simulink library "halin"  (R2021b)
settings: Solver=VariableStepAuto  StartTime=0.0  StopTime=10.0  RelTol=1e-3
undefined symbols (not defined in the file): KHAL_CAN1ABM1E2E_flg, KHAL_CAN1EPB1E2E_flg, KHAL_CAN1EPS1E2E_flg, KHAL_CAN1ESC1E2E_flg, KHAL_CAN1ESC5E2E_flg, KHAL_CAN3BMS1E2E_flg, KHAL_CAN3BMS6E2E_flg, KHAL_CAN3CCU1E2E_flg, KHAL_CAN3CCU2E2E_flg, KHAL_CAN3MCUNF1E2E_flg, KHAL_CAN3MCUNR1E2E_flg, KHAL_CAN3Shifter1E2E_flg, KHAL_CAN3Shifter2E2E_flg, KHAL_CAN6FCM2E2E_flg, KHAL_CAN6FCM4E2E_flg, TRUE
libraries: simulink x645, FVT_lib x207, hcu_lib x59
(part 1 of 23)
settings Model: Creator=13168  LastModifiedBy=FVT23033
settings SolverCC: AlgebraicLoopSolver=TrustRegion
settings DataIOCC: SaveFormat=Array  SignalLoggingSaveFormat=ModelDataLogs  ReturnWorkspaceOutputs=off
settings OptimizationCC: BlockReduction=off  BooleanDataType=off
settings DebuggingCC: SaveWithParameterizedLinksMsg=none  UnderspecifiedInitializationDetection=Classic  MergeDetectMultiDrivingBlocksExec=none  SignalResolutionControl=TryResolveAllWithWarning  SFMachineParentedDataDiag=warning
settings HardwareCC: TargetUnknown=on
settings ModelReferenceCC: PropagateSignalLabelsOutOfModel=off
settings ConfigComp: CovMetricSettings=dw  CovSaveCumulativeToWorkspaceVar=on  CovSaveSingleToWorkspaceVar=on

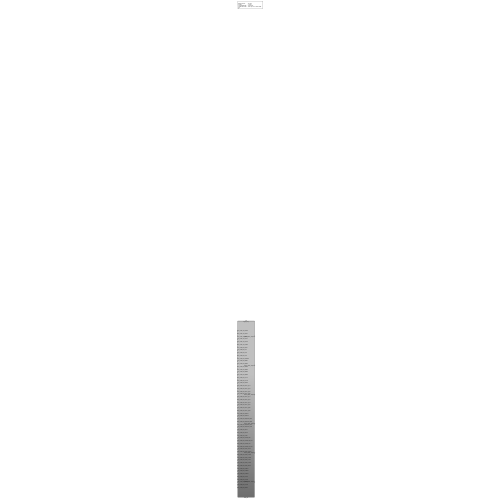
[thumbnail: Simulink's stored preview of the top-level diagram]
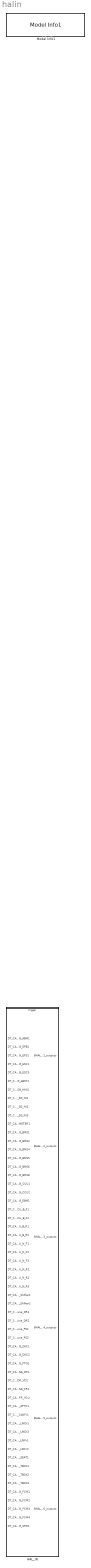
== system halin ==
  HAL_IN : Subsystem
      settings: RTWSystemCode=Nonreusable function  RTWFcnNameOpts=Use subsystem name  RTWFileNameOpts=Use subsystem name
  Model Info1 : hcu_lib/Model Info1  BlockCM=None  Frame=on  DisplayStringWithTags=|  HorizontalTextAlignment=Left  LeftAlignmentValue=0.02  SourceBlockDiagram=hcu_lib  TagMaxNumber=20
      | Model Version        : %<ModelVersion>
      | Creator                   : %<Creator>
      | Last Modified By    : %<LastModifiedBy>
      | Modification date    : %<LastModificationDate>
      settings: SourceProductName=HCU Relative Block Library

== system halin/HAL_IN ==
  DT_CAN1_SG_ABM1 : Inport
  DT_CAN1_SG_EPB1 : Inport  Port=2
  DT_CAN1_SG_EPS1 : Inport  Port=3
  DT_CAN1_SG_ESC1 : Inport  Port=4
  DT_CAN1_SG_ESC5 : Inport  Port=5
  DT_CAN1_SG_eBST1 : Inport  Port=6
  DT_CAN2_SG_HMI1 : Inport  Port=7
  DT_CAN2_SG_IVI1 : Inport  Port=8
  DT_CAN2_SG_IVI2 : Inport  Port=9
  DT_CAN2_SG_IVI3 : Inport  Port=10
  DT_CAN2_SG_METER1 : Inport  Port=11
  DT_CAN3_SG_BMS1 : Inport  Port=12
  DT_CAN3_SG_BMS3 : Inport  Port=13
  DT_CAN3_SG_BMS4 : Inport  Port=14
  DT_CAN3_SG_BMS5 : Inport  Port=15
  DT_CAN3_SG_BMS6 : Inport  Port=16
  DT_CAN3_SG_BMS8 : Inport  Port=17
  DT_CAN3_SG_CCU1 : Inport  Port=18
  DT_CAN3_SG_CCU2 : Inport  Port=19
  DT_CAN3_SG_EBM1 : Inport  Port=20
  DT_CAN3_SG_MCU_B_F1 : Inport  Port=21
  DT_CAN3_SG_MCU_B_F2 : Inport  Port=22
  DT_CAN3_SG_MCU_B_R1 : Inport  Port=23
  DT_CAN3_SG_MCU_B_R2 : Inport  Port=24
  DT_CAN3_SG_MCU_N_F1 : Inport  Port=25
  DT_CAN3_SG_MCU_N_F2 : Inport  Port=26
  DT_CAN3_SG_MCU_N_F3 : Inport  Port=27
  DT_CAN3_SG_MCU_N_R1 : Inport  Port=28
  DT_CAN3_SG_MCU_N_R2 : Inport  Port=29
  DT_CAN3_SG_MCU_N_R3 : Inport  Port=30
  DT_CAN3_SG_Shifter1 : Inport  Port=31
  DT_CAN3_SG_Shifter2 : Inport  Port=32
  DT_CAN4_SG_BodyZone_DR1 : Inport  Port=33
  DT_CAN4_SG_BodyZone_DR2 : Inport  Port=34
  DT_CAN4_SG_BodyZone_PS1 : Inport  Port=35
  DT_CAN4_SG_BodyZone_PS2 : Inport  Port=36
  DT_CAN4_SG_DKC1 : Inport  Port=37
  DT_CAN4_SG_DKC2 : Inport  Port=38
  DT_CAN4_SG_PTG1 : Inport  Port=39
  DT_CAN4_SG_ZONE_DR1 : Inport  Port=40
  DT_CAN4_SG_ZONE_DR_VCU : Inport  Port=41
  DT_CAN4_SG_ZONE_FR1 : Inport  Port=42
  DT_CAN4_SG_ZONE_FR_VCU : Inport  Port=43
  DT_CAN4_SG_zGW_APTC1 : Inport  Port=44
  DT_CAN4_SG_zGW_CANFr1 : Inport  Port=45
  DT_CAN4_SG_zGW_LINDr1 : Inport  Port=46
  DT_CAN4_SG_zGW_LINDr2 : Inport  Port=47
  DT_CAN4_SG_zGW_LINFr1 : Inport  Port=48
  DT_CAN4_SG_zGW_LINFr2 : Inport  Port=49
  DT_CAN4_SG_zGW_SEAT1 : Inport  Port=50
  DT_CAN5_SG_TBOX1 : Inport  Port=51
  DT_CAN5_SG_TBOX2 : Inport  Port=52
  DT_CAN5_SG_TBOX3 : Inport  Port=53
  DT_CAN6_SG_FCM1 : Inport  Port=54
  DT_CAN6_SG_FCM2 : Inport  Port=55
  DT_CAN6_SG_FCM3 : Inport  Port=56
  DT_CAN6_SG_FCM4 : Inport  Port=57
  DT_CAN6_SG_SRR1 : Inport  Port=58
  trig_hal_in : TriggerPort  TriggerType=function-call  VariantControl=(inherit)
  CAN1 : Subsystem
  CAN2 : Subsystem
  CAN3 : Subsystem
  CAN4 : Subsystem
  CAN5 : Subsystem
  CAN6 : Subsystem
  BHAL_CAN1_outputs : Outport  OutDataTypeStr=Bus: BHAL_CAN1_outputs
  BHAL_CAN2_outputs : Outport  Port=2  OutDataTypeStr=Bus: BHAL_CAN2_outputs
  BHAL_CAN3_outputs : Outport  Port=3  OutDataTypeStr=Bus: BHAL_CAN3_outputs
  BHAL_CAN4_outputs : Outport  Port=4  OutDataTypeStr=Bus: BHAL_CAN4_outputs
  BHAL_CAN5_outputs : Outport  Port=5  OutDataTypeStr=Bus: BHAL_CAN5_outputs
  BHAL_CAN6_outputs : Outport  Port=6  OutDataTypeStr=Bus: BHAL_CAN6_outputs
  wires:
  CAN1/1(HAL_CAN1_outputs) -> BHAL_CAN1_outputs/1
  DT_CAN1_SG_EPS1/1 -> CAN1/3(DT_CAN1_SG_EPS1)
  DT_CAN1_SG_EPB1/1 -> CAN1/2(DT_CAN1_SG_EPB1)
  DT_CAN2_SG_METER1/1 -> CAN2/5(DT_CAN2_SG_METER1)
  DT_CAN2_SG_IVI2/1 -> CAN2/3(DT_CAN2_SG_IVI2)
  DT_CAN1_SG_ABM1/1 -> CAN1/1(DT_CAN1_SG_ABM1)
  DT_CAN2_SG_HMI1/1 -> CAN2/1(DT_CAN2_SG_HMI1)
  CAN2/1(HAL_CAN2_outputs) -> BHAL_CAN2_outputs/1
  DT_CAN3_SG_EBM1/1 -> CAN3/9(DT_CAN3_SG_EBM1)
  DT_CAN3_SG_MCU_B_R1/1 -> CAN3/12(DT_CAN3_SG_MCU_B_R1)
  DT_CAN6_SG_FCM4/1 -> CAN6/4(DT_CAN6_SG_FCM4)
  DT_CAN6_SG_FCM2/1 -> CAN6/2(DT_CAN6_SG_FCM2)
  CAN6/1(HAL_CAN6_outputs) -> BHAL_CAN6_outputs/1
  DT_CAN5_SG_TBOX2/1 -> CAN5/2(DT_CAN5_SG_TBOX2)
  DT_CAN3_SG_CCU1/1 -> CAN3/7(DT_CAN3_SG_CCU1)
  DT_CAN4_SG_zGW_APTC1/1 -> CAN4/12(DT_CAN4_SG_zGW_APTC1)
  DT_CAN3_SG_CCU2/1 -> CAN3/8(DT_CAN3_SG_CCU2)
  DT_CAN4_SG_zGW_CANFr1/1 -> CAN4/13(DT_CAN4_SG_zGW_CANFr1)
  CAN5/1(HAL_CAN5_outputs) -> BHAL_CAN5_outputs/1
  DT_CAN4_SG_ZONE_DR_VCU/1 -> CAN4/9(DT_CAN4_SG_ZONE_DR_VCU)
  DT_CAN3_SG_Shifter2/1 -> CAN3/21(DT_CAN3_SG_Shifter2)
  DT_CAN3_SG_MCU_N_R2/1 -> CAN3/18(DT_CAN3_SG_MCU_N_R2)
  DT_CAN4_SG_zGW_LINDr1/1 -> CAN4/14(DT_CAN4_SG_zGW_LINDr1)
  DT_CAN3_SG_MCU_N_R3/1 -> CAN3/19(DT_CAN3_SG_MCU_N_R3)
  DT_CAN3_SG_MCU_N_R1/1 -> CAN3/17(DT_CAN3_SG_MCU_N_R1)
  DT_CAN2_SG_IVI3/1 -> CAN2/4(DT_CAN2_SG_IVI3)
  DT_CAN3_SG_MCU_N_F3/1 -> CAN3/16(DT_CAN3_SG_MCU_N_F3)
  DT_CAN3_SG_MCU_N_F1/1 -> CAN3/14(DT_CAN3_SG_MCU_N_F1)
  DT_CAN3_SG_MCU_N_F2/1 -> CAN3/15(DT_CAN3_SG_MCU_N_F2)
  DT_CAN6_SG_FCM1/1 -> CAN6/1(DT_CAN6_SG_FCM1)
  DT_CAN3_SG_MCU_B_R2/1 -> CAN3/13(DT_CAN3_SG_MCU_B_R2)
  DT_CAN6_SG_SRR1/1 -> CAN6/5(DT_CAN6_SG_SRR1)
  DT_CAN3_SG_MCU_B_F2/1 -> CAN3/11(DT_CAN3_SG_MCU_B_F2)
  DT_CAN5_SG_TBOX1/1 -> CAN5/1(DT_CAN5_SG_TBOX1)
  DT_CAN1_SG_eBST1/1 -> CAN1/6(DT_CAN1_SG_eBST1)
  DT_CAN4_SG_DKC2/1 -> CAN4/6(DT_CAN4_SG_DKC2)
  DT_CAN2_SG_IVI1/1 -> CAN2/2(DT_CAN2_SG_IVI1)
  DT_CAN4_SG_DKC1/1 -> CAN4/5(DT_CAN4_SG_DKC1)
  DT_CAN4_SG_BodyZone_DR2/1 -> CAN4/2(DT_CAN4_SG_BodyZone_DR2)
  DT_CAN4_SG_BodyZone_PS1/1 -> CAN4/3(DT_CAN4_SG_BodyZone_PS1)
  DT_CAN4_SG_BodyZone_DR1/1 -> CAN4/1(DT_CAN4_SG_BodyZone_DR1)
  DT_CAN4_SG_PTG1/1 -> CAN4/7(DT_CAN4_SG_PTG1)
  DT_CAN4_SG_zGW_LINDr2/1 -> CAN4/15(DT_CAN4_SG_zGW_LINDr2)
  DT_CAN5_SG_TBOX3/1 -> CAN5/3(DT_CAN5_SG_TBOX3)
  DT_CAN1_SG_ESC1/1 -> CAN1/4(DT_CAN1_SG_ESC1)
  DT_CAN3_SG_BMS8/1 -> CAN3/6(DT_CAN3_SG_BMS8)
  DT_CAN4_SG_BodyZone_PS2/1 -> CAN4/4(DT_CAN4_SG_BodyZone_PS2)
  DT_CAN3_SG_Shifter1/1 -> CAN3/20(DT_CAN3_SG_Shifter1)
  DT_CAN3_SG_BMS6/1 -> CAN3/5(DT_CAN3_SG_BMS6)
  DT_CAN3_SG_BMS4/1 -> CAN3/3(DT_CAN3_SG_BMS4)
  DT_CAN4_SG_ZONE_FR_VCU/1 -> CAN4/11(DT_CAN4_SG_ZONE_FR_VCU)
  DT_CAN1_SG_ESC5/1 -> CAN1/5(DT_CAN1_SG_ESC5)
  DT_CAN3_SG_BMS3/1 -> CAN3/2(DT_CAN3_SG_BMS3)
  DT_CAN3_SG_BMS1/1 -> CAN3/1(DT_CAN3_SG_BMS1)
  DT_CAN4_SG_ZONE_DR1/1 -> CAN4/8(DT_CAN4_SG_ZONE_DR1)
  CAN4/1(HAL_CAN4_outputs) -> BHAL_CAN4_outputs/1
  DT_CAN4_SG_zGW_SEAT1/1 -> CAN4/18(DT_CAN4_SG_zGW_SEAT1)
  DT_CAN3_SG_MCU_B_F1/1 -> CAN3/10(DT_CAN3_SG_MCU_B_F1)
  DT_CAN6_SG_FCM3/1 -> CAN6/3(DT_CAN6_SG_FCM3)
  DT_CAN4_SG_zGW_LINFr2/1 -> CAN4/17(DT_CAN4_SG_zGW_LINFr2)
  CAN3/1(HAL_CAN3_outputs) -> BHAL_CAN3_outputs/1
  DT_CAN3_SG_BMS5/1 -> CAN3/4(DT_CAN3_SG_BMS5)
  DT_CAN4_SG_ZONE_FR1/1 -> CAN4/10(DT_CAN4_SG_ZONE_FR1)
  DT_CAN4_SG_zGW_LINFr1/1 -> CAN4/16(DT_CAN4_SG_zGW_LINFr1)

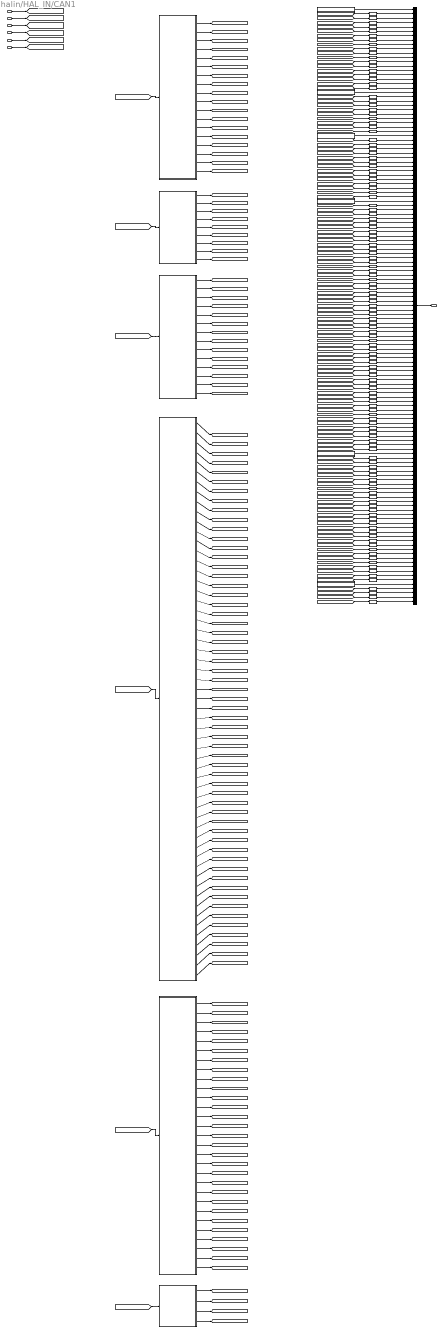
== system halin/HAL_IN/CAN1 ==
  DT_CAN1_SG_ABM1 : Inport
  DT_CAN1_SG_EPB1 : Inport  Port=2
  DT_CAN1_SG_EPS1 : Inport  Port=3
  DT_CAN1_SG_ESC1 : Inport  Port=4
  DT_CAN1_SG_ESC5 : Inport  Port=5
  DT_CAN1_SG_eBST1 : Inport  Port=6
  ABM1 : Subsystem
  EPB1 : Subsystem
  EPS1 : Subsystem
  ESC1 : Subsystem
  ESC5 : Subsystem
  UnitConverter{,1..6,9,11..20,22,24..25,27..28,32..34,37,39..51,54..56,58,60..61,64..69,71,73,76,78,80..81,83,85,88,90,93..96,98..103,105..107,112..113,116,118,120,124,126..130} (86 alike) : DataTypeConversion  OutDataTypeStr=boolean
  UnitConverter{7..8,10,21,23,26,29..31,35,52..53,57,59,70,74..75,79,82,86..87,91,108..111,122} (27 alike) : DataTypeConversion  OutDataTypeStr=uint8
  UnitConverter{36,38,62..63,72,77,84,89,92,97,104,114..115,117,119,121,123,125} (18 alike) : DataTypeConversion  OutDataTypeStr=single
  VHAL_CANMsgInvalidABM1_flg : Subsystem  AncestorBlock=FVT_lib/hal/MsgTimeoutJudge_CAN_AUTOSAR
      mask help: MeasumentTrigerEvent
      mask Display: fprintf('MsgTimeoutJudge_CAN\nAUTOSAR');
  VHAL_CANMsgInvalidEPB1_flg : Subsystem  AncestorBlock=FVT_lib/hal/MsgTimeoutJudge_CAN_AUTOSAR
      mask help: MeasumentTrigerEvent
      mask Display: fprintf('MsgTimeoutJudge_CAN\nAUTOSAR');
  VHAL_CANMsgInvalidEPS1_flg : Subsystem  AncestorBlock=FVT_lib/hal/MsgTimeoutJudge_CAN_AUTOSAR
      mask help: MeasumentTrigerEvent
      mask Display: fprintf('MsgTimeoutJudge_CAN\nAUTOSAR');
  VHAL_CANMsgInvalidESC1_flg : Subsystem  AncestorBlock=FVT_lib/hal/MsgTimeoutJudge_CAN_AUTOSAR
      mask help: MeasumentTrigerEvent
      mask Display: fprintf('MsgTimeoutJudge_CAN\nAUTOSAR');
  VHAL_CANMsgInvalidESC5_flg : Subsystem  AncestorBlock=FVT_lib/hal/MsgTimeoutJudge_CAN_AUTOSAR
      mask help: MeasumentTrigerEvent
      mask Display: fprintf('MsgTimeoutJudge_CAN\nAUTOSAR');
  VHAL_CANMsgInvalideBST1_flg : Subsystem  AncestorBlock=FVT_lib/hal/MsgTimeoutJudge_CAN_AUTOSAR
      mask help: MeasumentTrigerEvent
      mask Display: fprintf('MsgTimeoutJudge_CAN\nAUTOSAR');
  bus_creator : BusCreator  Inputs=137
  eBST1 : Subsystem
  HAL_CAN1_outputs : Outport
  wires:
  DT_CAN1_SG_ABM1/1 -> [DT_CAN1_SG_ABM1]
  DT_CAN1_SG_EPB1/1 -> [DT_CAN1_SG_EPB1]
  DT_CAN1_SG_EPS1/1 -> [DT_CAN1_SG_EPS1]
  DT_CAN1_SG_ESC1/1 -> [DT_CAN1_SG_ESC1]
  DT_CAN1_SG_ESC5/1 -> [DT_CAN1_SG_ESC5]
  DT_CAN1_SG_eBST1/1 -> [DT_CAN1_SG_eBST1]
  [DT_CAN1_SG_ABM1] -> ABM1/1(DT_CAN1_SG_ABM1)
  [DT_CAN1_SG_EPB1] -> EPB1/1(DT_CAN1_SG_EPB1)
  [DT_CAN1_SG_EPS1] -> EPS1/1(DT_CAN1_SG_EPS1)
  [DT_CAN1_SG_ESC1] -> ESC1/1(DT_CAN1_SG_ESC1)
  [DT_CAN1_SG_ESC5] -> ESC5/1(DT_CAN1_SG_ESC5)
  [DT_CAN1_SG_eBST1] -> eBST1/1(DT_CAN1_SG_eBST1)
  bus_creator/1 -> HAL_CAN1_outputs/1
  VHAL_CANMsgInvalidABM1_flg/1(Out) -> bus_creator/1
  ABM1/1(VHAL_ABM1CSErr_flg) -> [VHAL_ABM1CSErr_flg]
  UnitConverter/1 -> bus_creator/2  "VHAL_ABM1CSErr_flg"
  [VHAL_ABM1CSErr_flg] -> UnitConverter/1
  ABM1/2(VHAL_ABM1RCErr_flg) -> [VHAL_ABM1RCErr_flg]
  UnitConverter1/1 -> bus_creator/3  "VHAL_ABM1RCErr_flg"
  [VHAL_ABM1RCErr_flg] -> UnitConverter1/1
  ABM1/3(VHAL_ABMPassengerODSSta_flg) -> [VHAL_ABMPassengerODSSta_flg]
  UnitConverter2/1 -> bus_creator/4  "VHAL_ABMPassengerODSSta_flg"
  [VHAL_ABMPassengerODSSta_flg] -> UnitConverter2/1
  ABM1/4(VHAL_ABMRearPassengerCTRODSSta_flg) -> [VHAL_ABMRearPassengerCTRODSSta_flg]
  UnitConverter3/1 -> bus_creator/5  "VHAL_ABMRearPassengerCTRODSSta_flg"
  [VHAL_ABMRearPassengerCTRODSSta_flg] -> UnitConverter3/1
  ABM1/5(VHAL_ABMRearPassengerLHODSSta_flg) -> [VHAL_ABMRearPassengerLHODSSta_flg]
  UnitConverter4/1 -> bus_creator/6  "VHAL_ABMRearPassengerLHODSSta_flg"
  [VHAL_ABMRearPassengerLHODSSta_flg] -> UnitConverter4/1
  ABM1/6(VHAL_ABMRearPassengerRHODSSta_flg) -> [VHAL_ABMRearPassengerRHODSSta_flg]
  UnitConverter5/1 -> bus_creator/7  "VHAL_ABMRearPassengerRHODSSta_flg"
  [VHAL_ABMRearPassengerRHODSSta_flg] -> UnitConverter5/1
  ABM1/7(VHAL_AirBagFailCmd_flg) -> [VHAL_AirBagFailCmd_flg]
  UnitConverter6/1 -> bus_creator/8  "VHAL_AirBagFailCmd_flg"
  [VHAL_AirBagFailCmd_flg] -> UnitConverter6/1
  ABM1/8(VHAL_ChecksumABM1_enum) -> [VHAL_ChecksumABM1_enum]
  UnitConverter7/1 -> bus_creator/9  "VHAL_ChecksumABM1_enum"
  [VHAL_ChecksumABM1_enum] -> UnitConverter7/1
  ABM1/9(VHAL_CrashOutputSts_enum) -> [VHAL_CrashOutputSts_enum]
  UnitConverter8/1 -> bus_creator/10  "VHAL_CrashOutputSts_enum"
  [VHAL_CrashOutputSts_enum] -> UnitConverter8/1
  ABM1/10(VHAL_DriverSeatBeltCmd_flg) -> [VHAL_DriverSeatBeltCmd_flg]
  UnitConverter9/1 -> bus_creator/11  "VHAL_DriverSeatBeltCmd_flg"
  [VHAL_DriverSeatBeltCmd_flg] -> UnitConverter9/1
  ABM1/11(VHAL_LifeCountABM1_enum) -> [VHAL_LifeCountABM1_enum]
  UnitConverter10/1 -> bus_creator/12  "VHAL_LifeCountABM1_enum"
  [VHAL_LifeCountABM1_enum] -> UnitConverter10/1
  ABM1/12(VHAL_PABSwitchCmd_flg) -> [VHAL_PABSwitchCmd_flg]
  UnitConverter11/1 -> bus_creator/13  "VHAL_PABSwitchCmd_flg"
  [VHAL_PABSwitchCmd_flg] -> UnitConverter11/1
  ABM1/13(VHAL_PsngrSeatBeltCmd_flg) -> [VHAL_PsngrSeatBeltCmd_flg]
  UnitConverter12/1 -> bus_creator/14  "VHAL_PsngrSeatBeltCmd_flg"
  [VHAL_PsngrSeatBeltCmd_flg] -> UnitConverter12/1
  ABM1/14(VHAL_RCenterSeatBeltCmd_flg) -> [VHAL_RCenterSeatBeltCmd_flg]
  UnitConverter13/1 -> bus_creator/15  "VHAL_RCenterSeatBeltCmd_flg"
  [VHAL_RCenterSeatBeltCmd_flg] -> UnitConverter13/1
  ABM1/15(VHAL_RDriverSeatBeltCmd_flg) -> [VHAL_RDriverSeatBeltCmd_flg]
  UnitConverter14/1 -> bus_creator/16  "VHAL_RDriverSeatBeltCmd_flg"
  [VHAL_RDriverSeatBeltCmd_flg] -> UnitConverter14/1
  ABM1/16(VHAL_RPsngrSeatBeltCmd_flg) -> [VHAL_RPsngrSeatBeltCmd_flg]
  UnitConverter15/1 -> bus_creator/17  "VHAL_RPsngrSeatBeltCmd_flg"
  [VHAL_RPsngrSeatBeltCmd_flg] -> UnitConverter15/1
  ABM1/17(VHAL_TLHPsngrSeatBeltCmd_flg) -> [VHAL_TLHPsngrSeatBeltCmd_flg]
  UnitConverter16/1 -> bus_creator/18  "VHAL_TLHPsngrSeatBeltCmd_flg"
  [VHAL_TLHPsngrSeatBeltCmd_flg] -> UnitConverter16/1
  ABM1/18(VHAL_TRHPsngrSeatBeltCmd_flg) -> [VHAL_TRHPsngrSeatBeltCmd_flg]
  UnitConverter17/1 -> bus_creator/19  "VHAL_TRHPsngrSeatBeltCmd_flg"
  [VHAL_TRHPsngrSeatBeltCmd_flg] -> UnitConverter17/1
  VHAL_CANMsgInvalidEPB1_flg/1(Out) -> bus_creator/20
  EPB1/1(VHAL_EPB1CSErr_flg) -> [VHAL_EPB1CSErr_flg]
  UnitConverter18/1 -> bus_creator/21  "VHAL_EPB1CSErr_flg"
  [VHAL_EPB1CSErr_flg] -> UnitConverter18/1
  EPB1/2(VHAL_EPB1RCErr_flg) -> [VHAL_EPB1RCErr_flg]
  UnitConverter19/1 -> bus_creator/22  "VHAL_EPB1RCErr_flg"
  [VHAL_EPB1RCErr_flg] -> UnitConverter19/1
  EPB1/3(VHAL_DOASta_flg) -> [VHAL_DOASta_flg]
  UnitConverter20/1 -> bus_creator/23  "VHAL_DOASta_flg"
  [VHAL_DOASta_flg] -> UnitConverter20/1
  EPB1/4(VHAL_EPB1RC_enum) -> [VHAL_EPB1RC_enum]
  UnitConverter21/1 -> bus_creator/24  "VHAL_EPB1RC_enum"
  [VHAL_EPB1RC_enum] -> UnitConverter21/1
  EPB1/5(VHAL_EPBCarWashMode_flg) -> [VHAL_EPBCarWashMode_flg]
  UnitConverter22/1 -> bus_creator/25  "VHAL_EPBCarWashMode_flg"
  [VHAL_EPBCarWashMode_flg] -> UnitConverter22/1
  EPB1/6(VHAL_EPBErrSta_enum) -> [VHAL_EPBErrSta_enum]
  UnitConverter23/1 -> bus_creator/26  "VHAL_EPBErrSta_enum"
  [VHAL_EPBErrSta_enum] -> UnitConverter23/1
  EPB1/7(VHAL_EPBExtApplyAvail_flg) -> [VHAL_EPBExtApplyAvail_flg]
  UnitConverter24/1 -> bus_creator/27  "VHAL_EPBExtApplyAvail_flg"
  [VHAL_EPBExtApplyAvail_flg] -> UnitConverter24/1
  EPB1/8(VHAL_EPBExtReleaseAvail_flg) -> [VHAL_EPBExtReleaseAvail_flg]
  UnitConverter25/1 -> bus_creator/28  "VHAL_EPBExtReleaseAvail_flg"
  [VHAL_EPBExtReleaseAvail_flg] -> UnitConverter25/1
  EPB1/9(VHAL_EPBSta_enum) -> [VHAL_EPBSta_enum]
  UnitConverter26/1 -> bus_creator/29  "VHAL_EPBSta_enum"
  [VHAL_EPBSta_enum] -> UnitConverter26/1
  VHAL_CANMsgInvalidEPS1_flg/1(Out) -> bus_creator/30
  EPS1/1(VHAL_EPS1CSErr_flg) -> [VHAL_EPS1CSErr_flg]
  UnitConverter27/1 -> bus_creator/31  "VHAL_EPS1CSErr_flg"
  [VHAL_EPS1CSErr_flg] -> UnitConverter27/1
  EPS1/2(VHAL_EPS1RCErr_flg) -> [VHAL_EPS1RCErr_flg]
  UnitConverter28/1 -> bus_creator/32  "VHAL_EPS1RCErr_flg"
  [VHAL_EPS1RCErr_flg] -> UnitConverter28/1
  EPS1/3(VHAL_DriIntend_enum) -> [VHAL_DriIntend_enum]
  UnitConverter29/1 -> bus_creator/33  "VHAL_DriIntend_enum"
  [VHAL_DriIntend_enum] -> UnitConverter29/1
  EPS1/4(VHAL_EPSAOIControl_enum) -> [VHAL_EPSAOIControl_enum]
  UnitConverter30/1 -> bus_creator/34  "VHAL_EPSAOIControl_enum"
  [VHAL_EPSAOIControl_enum] -> UnitConverter30/1
  EPS1/5(VHAL_EPSRC_enum) -> [VHAL_EPSRC_enum]
  UnitConverter31/1 -> bus_creator/35  "VHAL_EPSRC_enum"
  [VHAL_EPSRC_enum] -> UnitConverter31/1
  EPS1/6(VHAL_EPSTOIActivation_flg) -> [VHAL_EPSTOIActivation_flg]
  UnitConverter32/1 -> bus_creator/36  "VHAL_EPSTOIActivation_flg"
  [VHAL_EPSTOIActivation_flg] -> UnitConverter32/1
  EPS1/7(VHAL_EPSTOIFault_flg) -> [VHAL_EPSTOIFault_flg]
  UnitConverter33/1 -> bus_creator/37  "VHAL_EPSTOIFault_flg"
  [VHAL_EPSTOIFault_flg] -> UnitConverter33/1
  EPS1/8(VHAL_EPSTOIUnavailable_flg) -> [VHAL_EPSTOIUnavailable_flg]
  UnitConverter34/1 -> bus_creator/38  "VHAL_EPSTOIUnavailable_flg"
  [VHAL_EPSTOIUnavailable_flg] -> UnitConverter34/1
  EPS1/9(VHAL_EpasFailed_enum) -> [VHAL_EpasFailed_enum]
  UnitConverter35/1 -> bus_creator/39  "VHAL_EpasFailed_enum"
  [VHAL_EpasFailed_enum] -> UnitConverter35/1
  EPS1/10(VHAL_SASAngle_Deg) -> [VHAL_SASAngle_Deg]
  UnitConverter36/1 -> bus_creator/40  "VHAL_SASAngle_Deg"
  [VHAL_SASAngle_Deg] -> UnitConverter36/1
  EPS1/11(VHAL_SASCAL_flg) -> [VHAL_SASCAL_flg]
  UnitConverter37/1 -> bus_creator/41  "VHAL_SASCAL_flg"
  [VHAL_SASCAL_flg] -> UnitConverter37/1
  EPS1/12(VHAL_SASSpeed_degps) -> [VHAL_SASSpeed_degps]
  UnitConverter38/1 -> bus_creator/42  "VHAL_SASSpeed_degps"
  [VHAL_SASSpeed_degps] -> UnitConverter38/1
  EPS1/13(VHAL_SASSpeedValid_flg) -> [VHAL_SASSpeedValid_flg]
  UnitConverter39/1 -> bus_creator/43  "VHAL_SASSpeedValid_flg"
  [VHAL_SASSpeedValid_flg] -> UnitConverter39/1
  EPS1/14(VHAL_SASV_flg) -> [VHAL_SASV_flg]
  UnitConverter40/1 -> bus_creator/44  "VHAL_SASV_flg"
  [VHAL_SASV_flg] -> UnitConverter40/1
  VHAL_CANMsgInvalidESC1_flg/1(Out) -> bus_creator/45
  ESC1/1(VHAL_ESC1CSErr_flg) -> [VHAL_ESC1CSErr_flg]
  UnitConverter41/1 -> bus_creator/46  "VHAL_ESC1CSErr_flg"
  [VHAL_ESC1CSErr_flg] -> UnitConverter41/1
  ESC1/2(VHAL_ESC1RCErr_flg) -> [VHAL_ESC1RCErr_flg]
  UnitConverter42/1 -> bus_creator/47  "VHAL_ESC1RCErr_flg"
  [VHAL_ESC1RCErr_flg] -> UnitConverter42/1
  ESC1/3(VHAL_ABSActive_flg) -> [VHAL_ABSActive_flg]
  UnitConverter43/1 -> bus_creator/48  "VHAL_ABSActive_flg"
  [VHAL_ABSActive_flg] -> UnitConverter43/1
  ESC1/4(VHAL_ABSFailed_flg) -> [VHAL_ABSFailed_flg]
  UnitConverter44/1 -> bus_creator/49  "VHAL_ABSFailed_flg"
  [VHAL_ABSFailed_flg] -> UnitConverter44/1
  ESC1/5(VHAL_ABSWnlmpSta_flg) -> [VHAL_ABSWnlmpSta_flg]
  UnitConverter45/1 -> bus_creator/50  "VHAL_ABSWnlmpSta_flg"
  [VHAL_ABSWnlmpSta_flg] -> UnitConverter45/1
  ESC1/6(VHAL_AVHActive_flg) -> [VHAL_AVHActive_flg]
  UnitConverter46/1 -> bus_creator/51  "VHAL_AVHActive_flg"
  [VHAL_AVHActive_flg] -> UnitConverter46/1
  ESC1/7(VHAL_AVHFailed_flg) -> [VHAL_AVHFailed_flg]
  UnitConverter47/1 -> bus_creator/52  "VHAL_AVHFailed_flg"
  [VHAL_AVHFailed_flg] -> UnitConverter47/1
  ESC1/8(VHAL_AmberWnlmpSta_flg) -> [VHAL_AmberWnlmpSta_flg]
  UnitConverter48/1 -> bus_creator/53  "VHAL_AmberWnlmpSta_flg"
  [VHAL_AmberWnlmpSta_flg] -> UnitConverter48/1
  ESC1/9(VHAL_BTCSActive_flg) -> [VHAL_BTCSActive_flg]
  UnitConverter49/1 -> bus_creator/54  "VHAL_BTCSActive_flg"
  [VHAL_BTCSActive_flg] -> UnitConverter49/1
  ESC1/10(VHAL_EBDActive_flg) -> [VHAL_EBDActive_flg]
  UnitConverter50/1 -> bus_creator/55  "VHAL_EBDActive_flg"
  [VHAL_EBDActive_flg] -> UnitConverter50/1
  ESC1/11(VHAL_EBDFailed_flg) -> [VHAL_EBDFailed_flg]
  UnitConverter51/1 -> bus_creator/56  "VHAL_EBDFailed_flg"
  [VHAL_EBDFailed_flg] -> UnitConverter51/1
  ESC1/12(VHAL_ESC1CS_enum) -> [VHAL_ESC1CS_enum]
  UnitConverter52/1 -> bus_creator/57  "VHAL_ESC1CS_enum"
  [VHAL_ESC1CS_enum] -> UnitConverter52/1
  ESC1/13(VHAL_ESC1RC_enum) -> [VHAL_ESC1RC_enum]
  UnitConverter53/1 -> bus_creator/58  "VHAL_ESC1RC_enum"
  [VHAL_ESC1RC_enum] -> UnitConverter53/1
  ESC1/14(VHAL_ESCActive_flg) -> [VHAL_ESCActive_flg]
  UnitConverter54/1 -> bus_creator/59  "VHAL_ESCActive_flg"
  [VHAL_ESCActive_flg] -> UnitConverter54/1
  ESC1/15(VHAL_ESCBeepReq_flg) -> [VHAL_ESCBeepReq_flg]
  UnitConverter55/1 -> bus_creator/60  "VHAL_ESCBeepReq_flg"
  [VHAL_ESCBeepReq_flg] -> UnitConverter55/1
  ESC1/16(VHAL_ESCFailed_flg) -> [VHAL_ESCFailed_flg]
  UnitConverter56/1 -> bus_creator/61  "VHAL_ESCFailed_flg"
  [VHAL_ESCFailed_flg] -> UnitConverter56/1
  ESC1/17(VHAL_ESCOFFStatus_enum) -> [VHAL_ESCOFFStatus_enum]
  UnitConverter57/1 -> bus_creator/62  "VHAL_ESCOFFStatus_enum"
  [VHAL_ESCOFFStatus_enum] -> UnitConverter57/1
  ESC1/18(VHAL_ESCOfflmpSta_flg) -> [VHAL_ESCOfflmpSta_flg]
  UnitConverter58/1 -> bus_creator/63  "VHAL_ESCOfflmpSta_flg"
  [VHAL_ESCOfflmpSta_flg] -> UnitConverter58/1
  ESC1/19(VHAL_ESCWnlmpSta_enum) -> [VHAL_ESCWnlmpSta_enum]
  UnitConverter59/1 -> bus_creator/64  "VHAL_ESCWnlmpSta_enum"
  [VHAL_ESCWnlmpSta_enum] -> UnitConverter59/1
  ESC1/20(VHAL_ESSActive_flg) -> [VHAL_ESSActive_flg]
  UnitConverter60/1 -> bus_creator/65  "VHAL_ESSActive_flg"
  [VHAL_ESSActive_flg] -> UnitConverter60/1
  ESC1/21(VHAL_FrPTCSActive_flg) -> [VHAL_FrPTCSActive_flg]
  UnitConverter61/1 -> bus_creator/66  "VHAL_FrPTCSActive_flg"
  [VHAL_FrPTCSActive_flg] -> UnitConverter61/1
  ESC1/22(VHAL_FrntAxlTrqReqDrv_Nm) -> [VHAL_FrntAxlTrqReqDrv_Nm]
  UnitConverter62/1 -> bus_creator/67  "VHAL_FrntAxlTrqReqDrv_Nm"
  [VHAL_FrntAxlTrqReqDrv_Nm] -> UnitConverter62/1
  ESC1/23(VHAL_GRADE_Deg) -> [VHAL_GRADE_Deg]
  UnitConverter63/1 -> bus_creator/68  "VHAL_GRADE_Deg"
  [VHAL_GRADE_Deg] -> UnitConverter63/1
  ESC1/24(VHAL_HBBActive_flg) -> [VHAL_HBBActive_flg]
  UnitConverter64/1 -> bus_creator/69  "VHAL_HBBActive_flg"
  [VHAL_HBBActive_flg] -> UnitConverter64/1
  ESC1/25(VHAL_HBBFailed_flg) -> [VHAL_HBBFailed_flg]
  UnitConverter65/1 -> bus_creator/70  "VHAL_HBBFailed_flg"
  [VHAL_HBBFailed_flg] -> UnitConverter65/1
  ESC1/26(VHAL_HDDActive_flg) -> [VHAL_HDDActive_flg]
  UnitConverter66/1 -> bus_creator/71  "VHAL_HDDActive_flg"
  [VHAL_HDDActive_flg] -> UnitConverter66/1
  ESC1/27(VHAL_HDDFailed_flg) -> [VHAL_HDDFailed_flg]
  UnitConverter67/1 -> bus_creator/72  "VHAL_HDDFailed_flg"
  [VHAL_HDDFailed_flg] -> UnitConverter67/1
  ESC1/28(VHAL_HSAActive_flg) -> [VHAL_HSAActive_flg]
  UnitConverter68/1 -> bus_creator/73  "VHAL_HSAActive_flg"
  [VHAL_HSAActive_flg] -> UnitConverter68/1
  ESC1/29(VHAL_HSAFailed_flg) -> [VHAL_HSAFailed_flg]
  UnitConverter69/1 -> bus_creator/74  "VHAL_HSAFailed_flg"
  [VHAL_HSAFailed_flg] -> UnitConverter69/1
  ESC1/30(VHAL_LFPulseCount_enum) -> [VHAL_LFPulseCount_enum]
  UnitConverter70/1 -> bus_creator/75  "VHAL_LFPulseCount_enum"
  [VHAL_LFPulseCount_enum] -> UnitConverter70/1
  ESC1/31(VHAL_LFPulseCountV_flg) -> [VHAL_LFPulseCountV_flg]
  UnitConverter71/1 -> bus_creator/76  "VHAL_LFPulseCountV_flg"
  [VHAL_LFPulseCountV_flg] -> UnitConverter71/1
  ESC1/32(VHAL_LFRawWhlSpeed_kph) -> [VHAL_LFRawWhlSpeed_kph]
  UnitConverter72/1 -> bus_creator/77  "VHAL_LFRawWhlSpeed_kph"
  [VHAL_LFRawWhlSpeed_kph] -> UnitConverter72/1
  ESC1/33(VHAL_LFRawWhlSpeedV_flg) -> [VHAL_LFRawWhlSpeedV_flg]
  UnitConverter73/1 -> bus_creator/78  "VHAL_LFRawWhlSpeedV_flg"
  [VHAL_LFRawWhlSpeedV_flg] -> UnitConverter73/1
  ESC1/34(VHAL_LFWhlRotDir_enum) -> [VHAL_LFWhlRotDir_enum]
  UnitConverter74/1 -> bus_creator/79  "VHAL_LFWhlRotDir_enum"
  [VHAL_LFWhlRotDir_enum] -> UnitConverter74/1
  ESC1/35(VHAL_LRPulseCount_enum) -> [VHAL_LRPulseCount_enum]
  UnitConverter75/1 -> bus_creator/80  "VHAL_LRPulseCount_enum"
  [VHAL_LRPulseCount_enum] -> UnitConverter75/1
  ESC1/36(VHAL_LRPulseCountV_flg) -> [VHAL_LRPulseCountV_flg]
  UnitConverter76/1 -> bus_creator/81  "VHAL_LRPulseCountV_flg"
  [VHAL_LRPulseCountV_flg] -> UnitConverter76/1
  ESC1/37(VHAL_LRRawWhlSpeed_kph) -> [VHAL_LRRawWhlSpeed_kph]
  UnitConverter77/1 -> bus_creator/82  "VHAL_LRRawWhlSpeed_kph"
  [VHAL_LRRawWhlSpeed_kph] -> UnitConverter77/1
  ESC1/38(VHAL_LRRawWhlSpeedV_flg) -> [VHAL_LRRawWhlSpeedV_flg]
  UnitConverter78/1 -> bus_creator/83  "VHAL_LRRawWhlSpeedV_flg"
  [VHAL_LRRawWhlSpeedV_flg] -> UnitConverter78/1
  ESC1/39(VHAL_LRWhlRotDir_enum) -> [VHAL_LRWhlRotDir_enum]
  UnitConverter79/1 -> bus_creator/84  "VHAL_LRWhlRotDir_enum"
  [VHAL_LRWhlRotDir_enum] -> UnitConverter79/1
  ESC1/40(VHAL_PBAActive_flg) -> [VHAL_PBAActive_flg]
  UnitConverter80/1 -> bus_creator/85  "VHAL_PBAActive_flg"
  [VHAL_PBAActive_flg] -> UnitConverter80/1
  ESC1/41(VHAL_PBAFailed_flg) -> [VHAL_PBAFailed_flg]
  UnitConverter81/1 -> bus_creator/86  "VHAL_PBAFailed_flg"
  [VHAL_PBAFailed_flg] -> UnitConverter81/1
  ESC1/42(VHAL_RFPulseCount_enum) -> [VHAL_RFPulseCount_enum]
  UnitConverter82/1 -> bus_creator/87  "VHAL_RFPulseCount_enum"
  [VHAL_RFPulseCount_enum] -> UnitConverter82/1
  ESC1/43(VHAL_RFPulseCountV_flg) -> [VHAL_RFPulseCountV_flg]
  UnitConverter83/1 -> bus_creator/88  "VHAL_RFPulseCountV_flg"
  [VHAL_RFPulseCountV_flg] -> UnitConverter83/1
  ESC1/44(VHAL_RFRawWhlSpeed_kph) -> [VHAL_RFRawWhlSpeed_kph]
  UnitConverter84/1 -> bus_creator/89  "VHAL_RFRawWhlSpeed_kph"
  [VHAL_RFRawWhlSpeed_kph] -> UnitConverter84/1
  ESC1/45(VHAL_RFRawWhlSpeedV_flg) -> [VHAL_RFRawWhlSpeedV_flg]
  UnitConverter85/1 -> bus_creator/90  "VHAL_RFRawWhlSpeedV_flg"
  [VHAL_RFRawWhlSpeedV_flg] -> UnitConverter85/1
  ESC1/46(VHAL_RFWhlRotDir_enum) -> [VHAL_RFWhlRotDir_enum]
  UnitConverter86/1 -> bus_creator/91  "VHAL_RFWhlRotDir_enum"
  [VHAL_RFWhlRotDir_enum] -> UnitConverter86/1
  ESC1/47(VHAL_RRPulseCount_enum) -> [VHAL_RRPulseCount_enum]
  UnitConverter87/1 -> bus_creator/92  "VHAL_RRPulseCount_enum"
  [VHAL_RRPulseCount_enum] -> UnitConverter87/1
  ESC1/48(VHAL_RRPulseCountV_flg) -> [VHAL_RRPulseCountV_flg]
  UnitConverter88/1 -> bus_creator/93  "VHAL_RRPulseCountV_flg"
  [VHAL_RRPulseCountV_flg] -> UnitConverter88/1
  ESC1/49(VHAL_RRRawWhlSpeed_kph) -> [VHAL_RRRawWhlSpeed_kph]
  UnitConverter89/1 -> bus_creator/94  "VHAL_RRRawWhlSpeed_kph"
  [VHAL_RRRawWhlSpeed_kph] -> UnitConverter89/1
  ESC1/50(VHAL_RRRawWhlSpeedV_flg) -> [VHAL_RRRawWhlSpeedV_flg]
  UnitConverter90/1 -> bus_creator/95  "VHAL_RRRawWhlSpeedV_flg"
  [VHAL_RRRawWhlSpeedV_flg] -> UnitConverter90/1
  ESC1/51(VHAL_RRWhlRotDir_enum) -> [VHAL_RRWhlRotDir_enum]
  UnitConverter91/1 -> bus_creator/96  "VHAL_RRWhlRotDir_enum"
  [VHAL_RRWhlRotDir_enum] -> UnitConverter91/1
  ESC1/52(VHAL_RearAxlTrqReqDrv_Nm) -> [VHAL_RearAxlTrqReqDrv_Nm]
  UnitConverter92/1 -> bus_creator/97  "VHAL_RearAxlTrqReqDrv_Nm"
  [VHAL_RearAxlTrqReqDrv_Nm] -> UnitConverter92/1
  ESC1/53(VHAL_RedWnlmpSta_flg) -> [VHAL_RedWnlmpSta_flg]
  UnitConverter93/1 -> bus_creator/98  "VHAL_RedWnlmpSta_flg"
  [VHAL_RedWnlmpSta_flg] -> UnitConverter93/1
  ESC1/54(VHAL_RrPTCSActive_flg) -> [VHAL_RrPTCSActive_flg]
  UnitConverter94/1 -> bus_creator/99  "VHAL_RrPTCSActive_flg"
  [VHAL_RrPTCSActive_flg] -> UnitConverter94/1
  ESC1/55(VHAL_TCSActive_flg) -> [VHAL_TCSActive_flg]
  UnitConverter95/1 -> bus_creator/100  "VHAL_TCSActive_flg"
  [VHAL_TCSActive_flg] -> UnitConverter95/1
  ESC1/56(VHAL_TCSFailed_flg) -> [VHAL_TCSFailed_flg]
  UnitConverter96/1 -> bus_creator/101  "VHAL_TCSFailed_flg"
  [VHAL_TCSFailed_flg] -> UnitConverter96/1
  ESC1/57(VHAL_VehSpeed_kph) -> [VHAL_VehSpeed_kph]
  UnitConverter97/1 -> bus_creator/102  "VHAL_VehSpeed_kph"
  [VHAL_VehSpeed_kph] -> UnitConverter97/1
  VHAL_CANMsgInvalidESC5_flg/1(Out) -> bus_creator/103
  ESC5/1(VHAL_ESC5CSErr_flg) -> [VHAL_ESC5CSErr_flg]
  UnitConverter98/1 -> bus_creator/104  "VHAL_ESC5CSErr_flg"
  [VHAL_ESC5CSErr_flg] -> UnitConverter98/1
  ESC5/2(VHAL_ESC5RCErr_flg) -> [VHAL_ESC5RCErr_flg]
  UnitConverter99/1 -> bus_creator/105  "VHAL_ESC5RCErr_flg"
  [VHAL_ESC5RCErr_flg] -> UnitConverter99/1
  ESC5/3(VHAL_ACCAvail_flg) -> [VHAL_ACCAvail_flg]
  UnitConverter100/1 -> bus_creator/106  "VHAL_ACCAvail_flg"
  [VHAL_ACCAvail_flg] -> UnitConverter100/1
  ESC5/4(VHAL_AEBAvail_flg) -> [VHAL_AEBAvail_flg]
  UnitConverter101/1 -> bus_creator/107  "VHAL_AEBAvail_flg"
  [VHAL_AEBAvail_flg] -> UnitConverter101/1
  ESC5/5(VHAL_ActBrkLampSta_flg) -> [VHAL_ActBrkLampSta_flg]
  UnitConverter102/1 -> bus_creator/108  "VHAL_ActBrkLampSta_flg"
  [VHAL_ActBrkLampSta_flg] -> UnitConverter102/1
  ESC5/6(VHAL_BrkDiscTempSta_flg) -> [VHAL_BrkDiscTempSta_flg]
  UnitConverter103/1 -> bus_creator/109  "VHAL_BrkDiscTempSta_flg"
  [VHAL_BrkDiscTempSta_flg] -> UnitConverter103/1
  ESC5/7(VHAL_BrkPedalPos_pct) -> [VHAL_BrkPedalPos_pct]
  UnitConverter104/1 -> bus_creator/110  "VHAL_BrkPedalPos_pct"
  [VHAL_BrkPedalPos_pct] -> UnitConverter104/1
  ESC5/8(VHAL_BrkPedalPosSta_flg) -> [VHAL_BrkPedalPosSta_flg]
  UnitConverter105/1 -> bus_creator/111  "VHAL_BrkPedalPosSta_flg"
  [VHAL_BrkPedalPosSta_flg] -> UnitConverter105/1
  ESC5/9(VHAL_BrkSwSta_flg) -> [VHAL_BrkSwSta_flg]
  UnitConverter106/1 -> bus_creator/112  "VHAL_BrkSwSta_flg"
  [VHAL_BrkSwSta_flg] -> UnitConverter106/1
  ESC5/10(VHAL_BrkSwV_flg) -> [VHAL_BrkSwV_flg]
  UnitConverter107/1 -> bus_creator/113  "VHAL_BrkSwV_flg"
  [VHAL_BrkSwV_flg] -> UnitConverter107/1
  ESC5/11(VHAL_ESC5CS_enum) -> [VHAL_ESC5CS_enum]
  UnitConverter108/1 -> bus_creator/114  "VHAL_ESC5CS_enum"
  [VHAL_ESC5CS_enum] -> UnitConverter108/1
  ESC5/12(VHAL_ESC5RC_enum) -> [VHAL_ESC5RC_enum]
  UnitConverter109/1 -> bus_creator/115  "VHAL_ESC5RC_enum"
  [VHAL_ESC5RC_enum] -> UnitConverter109/1
  ESC5/13(VHAL_ESCADASSta_enum) -> [VHAL_ESCADASSta_enum]
  UnitConverter110/1 -> bus_creator/116  "VHAL_ESCADASSta_enum"
  [VHAL_ESCADASSta_enum] -> UnitConverter110/1
  ESC5/14(VHAL_ESCAPSSta_enum) -> [VHAL_ESCAPSSta_enum]
  UnitConverter111/1 -> bus_creator/117  "VHAL_ESCAPSSta_enum"
  [VHAL_ESCAPSSta_enum] -> UnitConverter111/1
  ESC5/15(VHAL_ESCStandstill_flg) -> [VHAL_ESCStandstill_flg]
  UnitConverter112/1 -> bus_creator/118  "VHAL_ESCStandstill_flg"
  [VHAL_ESCStandstill_flg] -> UnitConverter112/1
  ESC5/16(VHAL_FrRBCActive_flg) -> [VHAL_FrRBCActive_flg]
  UnitConverter113/1 -> bus_creator/119  "VHAL_FrRBCActive_flg"
  [VHAL_FrRBCActive_flg] -> UnitConverter113/1
  ESC5/17(VHAL_FrntAxlTrqReqBrk_Nm) -> [VHAL_FrntAxlTrqReqBrk_Nm]
  UnitConverter114/1 -> bus_creator/120  "VHAL_FrntAxlTrqReqBrk_Nm"
  [VHAL_FrntAxlTrqReqBrk_Nm] -> UnitConverter114/1
  ESC5/18(VHAL_LatAccel_Gps) -> [VHAL_LatAccel_Gps]
  UnitConverter115/1 -> bus_creator/121  "VHAL_LatAccel_Gps"
  [VHAL_LatAccel_Gps] -> UnitConverter115/1
  ESC5/19(VHAL_LatAccelV_flg) -> [VHAL_LatAccelV_flg]
  UnitConverter116/1 -> bus_creator/122  "VHAL_LatAccelV_flg"
  [VHAL_LatAccelV_flg] -> UnitConverter116/1
  ESC5/20(VHAL_LongAccel_Gps) -> [VHAL_LongAccel_Gps]
  UnitConverter117/1 -> bus_creator/123  "VHAL_LongAccel_Gps"
  [VHAL_LongAccel_Gps] -> UnitConverter117/1
  ESC5/21(VHAL_LongAccelV_flg) -> [VHAL_LongAccelV_flg]
  UnitConverter118/1 -> bus_creator/124  "VHAL_LongAccelV_flg"
  [VHAL_LongAccelV_flg] -> UnitConverter118/1
  ESC5/22(VHAL_MCPressure_bar) -> [VHAL_MCPressure_bar]
  UnitConverter119/1 -> bus_creator/125  "VHAL_MCPressure_bar"
  [VHAL_MCPressure_bar] -> UnitConverter119/1
  ESC5/23(VHAL_MCPressureV_flg) -> [VHAL_MCPressureV_flg]
  UnitConverter120/1 -> bus_creator/126  "VHAL_MCPressureV_flg"
  [VHAL_MCPressureV_flg] -> UnitConverter120/1
  ESC5/24(VHAL_MeterIndVehSpeed_kph) -> [VHAL_MeterIndVehSpeed_kph]
  UnitConverter121/1 -> bus_creator/127  "VHAL_MeterIndVehSpeed_kph"
  [VHAL_MeterIndVehSpeed_kph] -> UnitConverter121/1
  ESC5/25(VHAL_RDCActive_enum) -> [VHAL_RDCActive_enum]
  UnitConverter122/1 -> bus_creator/128  "VHAL_RDCActive_enum"
  [VHAL_RDCActive_enum] -> UnitConverter122/1
  ESC5/26(VHAL_RearAxlTrqReqBrk_Nm) -> [VHAL_RearAxlTrqReqBrk_Nm]
  UnitConverter123/1 -> bus_creator/129  "VHAL_RearAxlTrqReqBrk_Nm"
  [VHAL_RearAxlTrqReqBrk_Nm] -> UnitConverter123/1
  ESC5/27(VHAL_RrRBCActive_flg) -> [VHAL_RrRBCActive_flg]
  UnitConverter124/1 -> bus_creator/130  "VHAL_RrRBCActive_flg"
  [VHAL_RrRBCActive_flg] -> UnitConverter124/1
  ESC5/28(VHAL_YawRate_degps) -> [VHAL_YawRate_degps]
  UnitConverter125/1 -> bus_creator/131  "VHAL_YawRate_degps"
  [VHAL_YawRate_degps] -> UnitConverter125/1
  ESC5/29(VHAL_YawRateV_flg) -> [VHAL_YawRateV_flg]
  UnitConverter126/1 -> bus_creator/132  "VHAL_YawRateV_flg"
  [VHAL_YawRateV_flg] -> UnitConverter126/1
  VHAL_CANMsgInvalideBST1_flg/1(Out) -> bus_creator/133
  eBST1/1(VHAL_LowBrakeFluidSta_flg) -> [VHAL_LowBrakeFluidSta_flg]
  UnitConverter127/1 -> bus_creator/134  "VHAL_LowBrakeFluidSta_flg"
  [VHAL_LowBrakeFluidSta_flg] -> UnitConverter127/1
  eBST1/2(VHAL_eBSTAmberWnlmpSta_flg) -> [VHAL_eBSTAmberWnlmpSta_flg]
  UnitConverter128/1 -> bus_creator/135  "VHAL_eBSTAmberWnlmpSta_flg"
  [VHAL_eBSTAmberWnlmpSta_flg] -> UnitConverter128/1
  eBST1/3(VHAL_eBSTBeepReq_flg) -> [VHAL_eBSTBeepReq_flg]
  UnitConverter129/1 -> bus_creator/136  "VHAL_eBSTBeepReq_flg"
  [VHAL_eBSTBeepReq_flg] -> UnitConverter129/1
  eBST1/4(VHAL_eBSTRedWnlmpSta_flg) -> [VHAL_eBSTRedWnlmpSta_flg]
  UnitConverter130/1 -> bus_creator/137  "VHAL_eBSTRedWnlmpSta_flg"
  [VHAL_eBSTRedWnlmpSta_flg] -> UnitConverter130/1
